simulink model "Quat_Mexp_Wertz"  (Simulink 7.5)
settings: Solver=ode45  StartTime=0.0  StopTime=10.0  RelTol=1e-3
values from neighbouring files (symbols this model uses):
  apSampleTime = 0.01    [demoz2SlugsV5.m]
  SampleT = 0.02    [demoz2SlugsV5.m]
libraries: dspmtrx3 x1
settings Model: Creator=Robert  LastModifiedBy=Robert

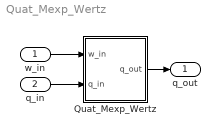
== system Quat_Mexp_Wertz ==
  w_in : Inport  OutDataType=fixdt(1, 16)  OutScaling=2^0
  q_in : Inport  Port=2  OutDataType=fixdt(1, 16)  OutScaling=2^0
  Quat_Mexp_Wertz : Subsystem
  q_out : Outport  OutDataType=fixdt(1, 16)  OutScaling=2^0
  wires:
  w_in/1 -> Quat_Mexp_Wertz/1(w_in)
  Quat_Mexp_Wertz/1(q_out) -> q_out/1
  q_in/1 -> Quat_Mexp_Wertz/2(q_in)

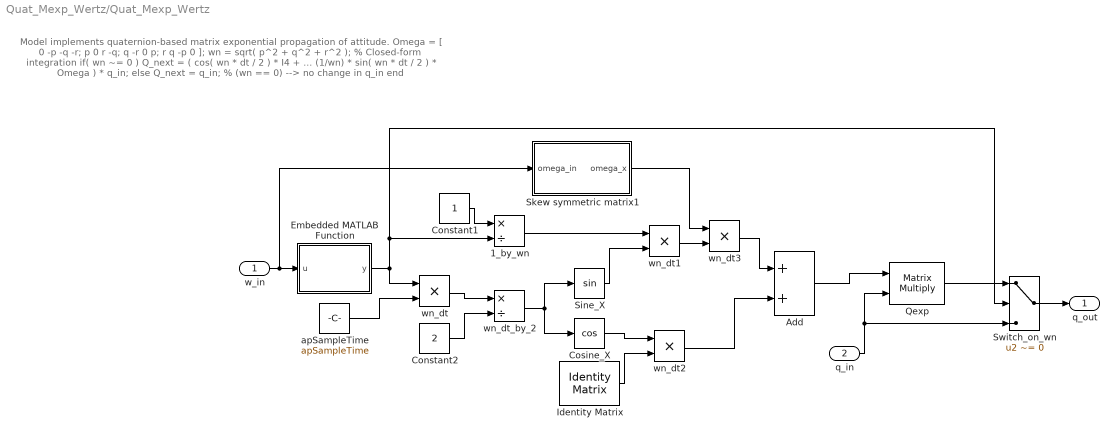
== system Quat_Mexp_Wertz/Quat_Mexp_Wertz ==
  note: Model implements quaternion-based matrix exponential propagation of attitude.
      | Omega = [ 0 -p -q -r; p 0 r -q; q -r 0 p; r q -p 0 ];
      | wn = sqrt( p^2 + q^2 + r^2 );
      |
      | % Closed-form integration
      | if( wn ~= 0 )
      |     Q_next = (   cos( wn * dt / 2 ) * I4 + ...
      |         (1/wn) * sin( wn * dt / 2 ) * Omega ) * q_in;
      | else
      |     Q_next = q_in; % (wn == 0) --> no change in q_in
      | end
  w_in : Inport  OutDataType=fixdt(1, 16)  OutScaling=2^0
  q_in : Inport  Port=2  OutDataType=fixdt(1, 16)  OutScaling=2^0
  1_by_wn : Product  Inputs=*/  OutDataType=fixdt(1, 16)  OutScaling=2^-10
  Add : Sum  OutDataTypeMode=single  OutDataType=fixdt(1, 16)  OutScaling=2^-10  OutDataTypeStr=single  SampleTime=apSampleTime
  Constant1 : Constant  OutDataTypeMode=single  OutDataType=fixdt(1, 16)  OutScaling=2^0  OutDataTypeStr=single
  Constant2 : Constant  Value=2  OutDataTypeMode=single  OutDataType=fixdt(1, 16)  OutScaling=2^0  OutDataTypeStr=single
  Cosine_X : Trigonometry  Operator=cos
  Embedded MATLAB Function : Stateflow chart  TreatAsAtomicUnit=on
  Identity Matrix : dspmtrx3/Identity Matrix  Inherit=off  N=4  Ts=apSampleTime  dataType=single  isSigned=on  wordLen=16  udDataType=sfix(16)  fracBitsMode=Best precision  numFracBits=15
  Qexp : Product  Multiplication=Matrix(*)  OutDataTypeMode=single  OutDataType=sfix(16)  OutScaling=2^0  OutDataTypeStr=single  SampleTime=SampleT
  Sine_X : Trigonometry
  Skew symmetric matrix1 : Subsystem
  Switch_on_wn : Switch  Criteria=u2 ~= 0  OutDataTypeMode=single  OutDataType=fixdt(1, 16)  OutScaling=2^0  OutDataTypeStr=single
  apSampleTime : Constant  Value=apSampleTime  OutDataTypeMode=single  OutDataType=fixdt(1, 16)  OutScaling=2^0  OutDataTypeStr=single
  wn_dt{,1..3} (4 alike) : Product  OutDataType=fixdt(1, 16)  OutScaling=2^0  RndMeth=Zero
  wn_dt_by_2 : Product  Inputs=*/  OutDataType=fixdt(1, 16)  OutScaling=2^-10
  q_out : Outport  OutDataType=fixdt(1, 16)  OutScaling=2^0
  wires:
  Embedded MATLAB Function/1(y) -> wn_dt/1, 1_by_wn/2, Switch_on_wn/2
  apSampleTime/1 -> wn_dt/2
  w_in/1 -> Embedded MATLAB Function/1(u), Skew symmetric matrix1/1(omega_in)
  wn_dt/1 -> wn_dt_by_2/1
  Constant2/1 -> wn_dt_by_2/2
  wn_dt_by_2/1 -> Sine_X/1, Cosine_X/1
  Constant1/1 -> 1_by_wn/1
  Sine_X/1 -> wn_dt1/2
  1_by_wn/1 -> wn_dt1/1
  wn_dt1/1 -> wn_dt3/2
  wn_dt3/1 -> Add/1
  Cosine_X/1 -> wn_dt2/1
  Identity Matrix/1 -> wn_dt2/2
  wn_dt2/1 -> Add/2
  Skew symmetric matrix1/1(omega_x) -> wn_dt3/1
  Qexp/1 -> Switch_on_wn/1
  Add/1 -> Qexp/1
  q_in/1 -> Qexp/2, Switch_on_wn/3
  Switch_on_wn/1 -> q_out/1

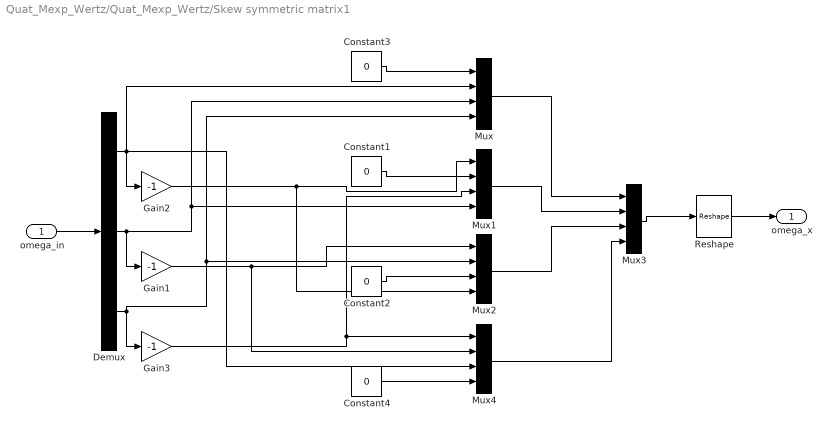
== system Quat_Mexp_Wertz/Quat_Mexp_Wertz/Skew symmetric matrix1 ==
  omega_in : Inport  DataType=single  OutDataType=fixdt(1, 16)  OutScaling=2^0  OutDataTypeStr=single
  Constant{1..4} (4 alike) : Constant  Value=0  OutDataTypeMode=single  OutDataType=fixdt(1, 16)  OutScaling=2^0  OutDataTypeStr=single
  Demux : Demux  Outputs=3
  Gain1 : Gain  Gain=-1  ParameterDataType=fixdt(1, 16)  ParameterScaling=2^0  OutDataTypeMode=single  OutDataType=fixdt(1, 16)  OutScaling=2^0  OutDataTypeStr=single
  Gain2 : Gain  Gain=-1  ParameterDataType=fixdt(1, 16)  ParameterScaling=2^0  OutDataTypeMode=single  OutDataType=fixdt(1, 16)  OutScaling=2^0  OutDataTypeStr=single
  Gain3 : Gain  Gain=-1  ParameterDataType=fixdt(1, 16)  ParameterScaling=2^0  OutDataTypeMode=single  OutDataType=fixdt(1, 16)  OutScaling=2^0  OutDataTypeStr=single
  Mux{,1..4} (5 alike) : Mux
  Reshape : Reshape  OutputDimensionality=Customize  OutputDimensions=[4,4]
  omega_x : Outport  DataType=single  OutDataType=fixdt(1, 16)  OutScaling=2^0  OutDataTypeStr=single
  wires:
  Demux/3 -> Gain3/1, Mux/4, Mux2/2
  Demux/2 -> Gain1/1, Mux/3, Mux1/4
  Demux/1 -> Gain2/1, Mux/2, Mux4/3
  Constant3/1 -> Mux/1
  Constant1/1 -> Mux1/2
  Constant2/1 -> Mux2/3
  Constant4/1 -> Mux4/4
  Mux4/1 -> Mux3/4
  Mux2/1 -> Mux3/3
  Mux1/1 -> Mux3/2
  Mux/1 -> Mux3/1
  omega_in/1 -> Demux/1
  Reshape/1 -> omega_x/1
  Mux3/1 -> Reshape/1
  Gain2/1 -> Mux1/1, Mux2/4
  Gain3/1 -> Mux1/3, Mux4/1
  Gain1/1 -> Mux2/1, Mux4/2

== matlab function Quat_Mexp_Wertz/Embedded MATLAB Function ==
  data: u input double; y output double
function y = GetNorm(u)
%#eml
% Function returns the 2-norm of the input argument.

y = norm(u);
